simulink model "ANCwithError"  (R2023b)
settings: Solver=VariableStepAuto  StartTime=0.0  StopTime=10.0  RelTol=1e-3
libraries: matrix_library x54, dspadpt3 x30, raspberrypiAVlib x2, dspfdesign x2, audiosources x1
(part 1 of 2)
settings Model: Creator=aaron  LastModifiedBy=aaron

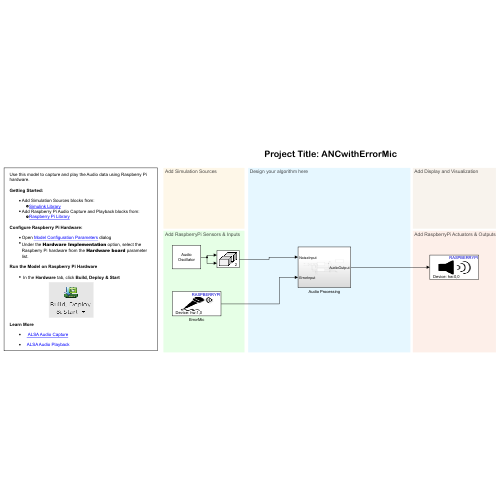
[thumbnail: Simulink's stored preview of the top-level diagram]
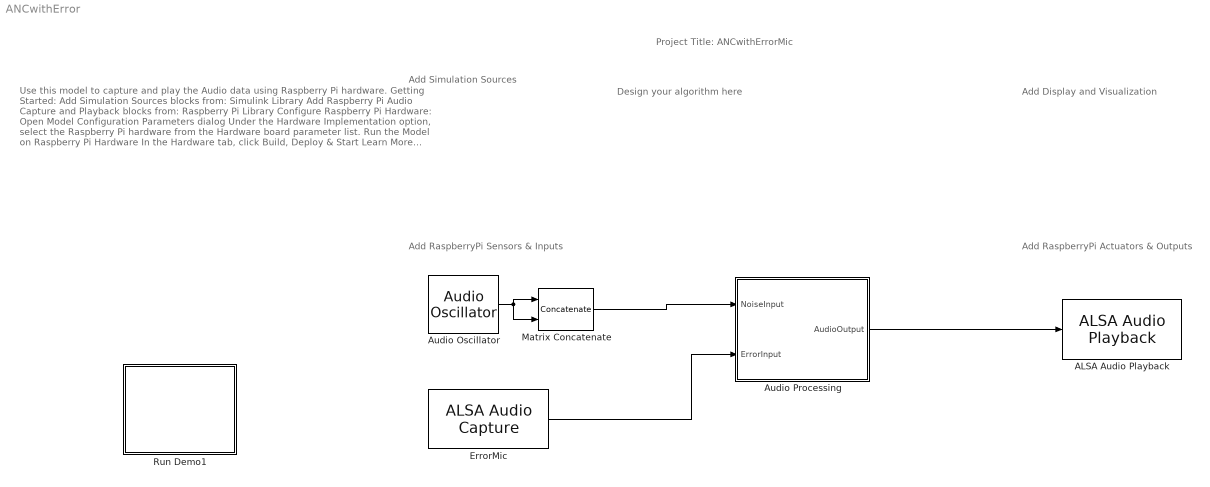
== system ANCwithError ==
  note: Use this model to capture and play the Audio data using Raspberry Pi hardware.
      |
      | Getting Started:
      |
      | Add Simulation Sources blocks from:
      | Simulink Library
      | Add Raspberry Pi Audio Capture and Playback blocks from:
      | Raspberry Pi Library
      |
      | Configure Raspberry Pi Hardware:
      |
      | Open Model Configuration Parameters dialog
      | Under the Hardware Implementation option, select the Raspberry Pi hardware from the Hardware board parameter list.
      |
      | Run the Model on Raspberry Pi Hardware
      |
      | In the Hardware tab, click Build, Deploy & Start
      |
      | Learn More
      | ALSA Audio Capture
      | ALSA Audio Playback
  note: Add Simulation Sources
  note: Add RaspberryPi Sensors & Inputs
  note: Project Title: ANCwithErrorMic
  note: Add Display and Visualization
  note: Add RaspberryPi Actuators & Outputs
  note: Design your algorithm here
  ALSA Audio Playback : raspberrypiAVlib/ALSA Audio Playback  deviceStr='hw:0,0'  sampleRateEnum=44100  queueDuration=0.5  blockPlatform=Raspberry Pi
  Audio Oscillator : audiosources/Audio Oscillator  FrequencyPort=off  Frequency=300  AmplitudePort=off  Amplitude=30000  DCOffsetPort=off  PhaseOffset=0  DCOffset=0  WidthPort=off  Width=1  DutyCyclePort=off  DutyCycle=0.5  SampsPerFrame=10  Fs=44100  OutputDataType=double  SimulateUsing=Code generation
      settings: SignalType=sine
  Audio Processing : Subsystem
  ErrorMic : raspberrypiAVlib/ALSA Audio Capture  deviceStr='hw:1,0'  DataBitDepth=16-bit integer  numberOfChannels=2  sampleRateEnum=44100  frameSize=SpF  QueueDuration=0.5  blockPlatform=Raspberry Pi
  Matrix Concatenate : Concatenate  Mode=Multidimensional array  ConcatenateDimension=2
  Run Demo1 : Subsystem  Description=Controls host-side RTDX processing.
      mask Display: pic=imread('raspberrypiBuildDeployAndStart.png');image(pic);
  wires:
  Matrix Concatenate/1 -> Audio Processing/1(NoiseInput)
  Audio Processing/1(AudioOutput) -> ALSA Audio Playback/1
  Audio Oscillator/1 -> Matrix Concatenate/2, Matrix Concatenate/1
  ErrorMic/1 -> Audio Processing/2(ErrorInput)

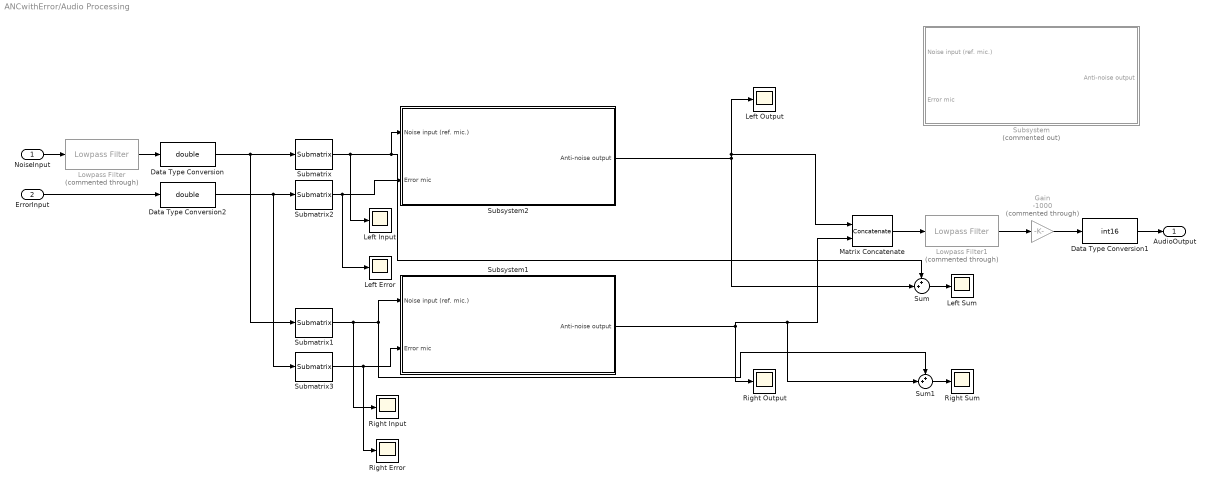
== system ANCwithError/Audio Processing ==
  NoiseInput : Inport
  ErrorInput : Inport  Port=2
  Data Type Conversion : DataTypeConversion  OutDataTypeStr=double  SaturateOnIntegerOverflow=off  RndMeth=Floor
  Data Type Conversion1 : DataTypeConversion  OutDataTypeStr=int16  SaturateOnIntegerOverflow=off  RndMeth=Floor  LockScale=on
  Data Type Conversion2 : DataTypeConversion  OutDataTypeStr=double  SaturateOnIntegerOverflow=off  RndMeth=Floor
  Gain : Gain  Commented=through  Gain=-1000
  Left Error : Scope
  Left Input : Scope
  Left Output : Scope
  Left Sum : Scope
  Lowpass Filter : dspfdesign/Lowpass Filter  Commented=through  FilterType=FIR  DesignForMinimumOrder=on  FilterOrder=50  PassbandFrequency=6e2  StopbandFrequency=10e2  PassbandRipple=0.1  StopbandAttenuation=80  SampleRateMode=Specify on dialog  SampleRate=44100  SimulateUsing=Interpreted execution  roundingMode=Floor  coeffsDataTypeStr=fixdt(1,16)
  Lowpass Filter1 : dspfdesign/Lowpass Filter  Commented=through  FilterType=FIR  DesignForMinimumOrder=on  FilterOrder=50  PassbandFrequency=6e2  StopbandFrequency=10e2  PassbandRipple=0.1  StopbandAttenuation=80  SampleRateMode=Specify on dialog  SampleRate=44100  SimulateUsing=Interpreted execution  roundingMode=Floor  coeffsDataTypeStr=fixdt(1,16)
  Matrix Concatenate : Concatenate  Mode=Multidimensional array  ConcatenateDimension=2
  Right Error : Scope
  Right Input : Scope
  Right Output : Scope
  Right Sum : Scope
  Submatrix : matrix_library/Submatrix  RowSpan=All rows  RowStartMode=First  RowStartIndex=1  RowEndMode=Last  RowEndIndex=1  ColSpan=One column  ColStartMode=First  ColStartIndex=1  ColEndMode=Last  ColEndIndex=1
  Submatrix1 : matrix_library/Submatrix  RowSpan=All rows  RowStartMode=First  RowStartIndex=1  RowEndMode=Last  RowEndIndex=1  ColSpan=One column  ColStartMode=Last  ColStartIndex=1  ColEndMode=Last  ColEndIndex=1
  Submatrix2 : matrix_library/Submatrix  RowSpan=All rows  RowStartMode=First  RowStartIndex=1  RowEndMode=Last  RowEndIndex=1  ColSpan=One column  ColStartMode=First  ColStartIndex=1  ColEndMode=Last  ColEndIndex=1
  Submatrix3 : matrix_library/Submatrix  RowSpan=All rows  RowStartMode=First  RowStartIndex=1  RowEndMode=Last  RowEndIndex=1  ColSpan=One column  ColStartMode=Last  ColStartIndex=1  ColEndMode=Last  ColEndIndex=1
  Subsystem : Subsystem  Commented=on  TreatAsAtomicUnit=on
  Subsystem1 : Subsystem  TreatAsAtomicUnit=on
  Subsystem2 : Subsystem  TreatAsAtomicUnit=on
  Sum : Sum  Inputs=++|
  Sum1 : Sum  Inputs=++|
  AudioOutput : Outport
  wires:
  Data Type Conversion/1 -> Submatrix1/1, Submatrix/1
  Submatrix/1 -> Subsystem2/1(Noise input (ref. mic.)), Sum/1, Left Input/1
  NoiseInput/1 -> Lowpass Filter/1
  Submatrix1/1 -> Sum1/1, Subsystem1/1(Noise input (ref. mic.)), Right Input/1
  Subsystem1/1(Anti-noise output) -> Sum1/2, Matrix Concatenate/2, Right Output/1
  Lowpass Filter/1 -> Data Type Conversion/1
  Gain/1 -> Data Type Conversion1/1
  Lowpass Filter1/1 -> Gain/1
  Data Type Conversion1/1 -> AudioOutput/1
  Matrix Concatenate/1 -> Lowpass Filter1/1
  Sum1/1 -> Right Sum/1
  Subsystem2/1(Anti-noise output) -> Left Output/1, Matrix Concatenate/1, Sum/2
  Sum/1 -> Left Sum/1
  ErrorInput/1 -> Data Type Conversion2/1
  Data Type Conversion2/1 -> Submatrix3/1, Submatrix2/1
  Submatrix2/1 -> Left Error/1, Subsystem2/2(Error mic)
  Submatrix3/1 -> Right Error/1, Subsystem1/2(Error mic)

== system ANCwithError/Run Demo1 ==

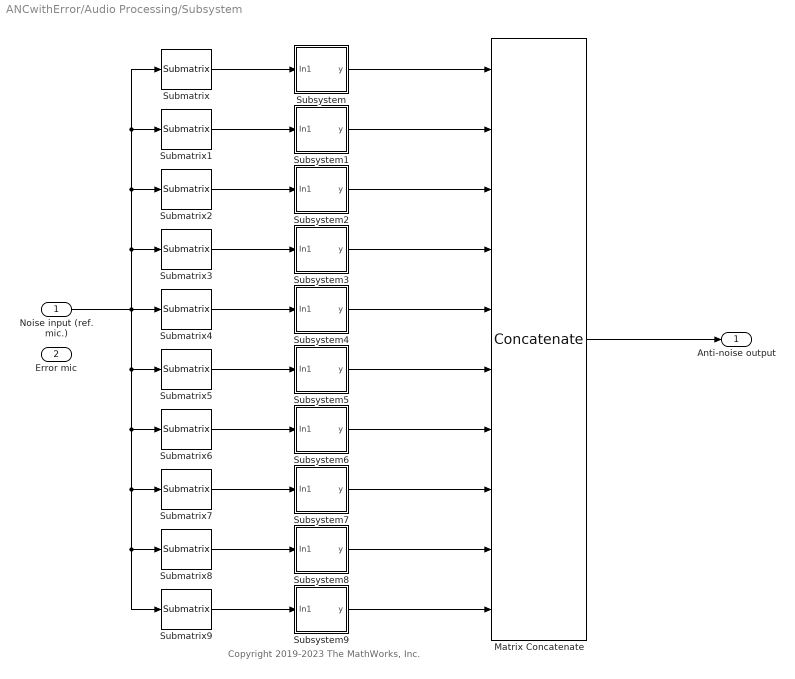
== system ANCwithError/Audio Processing/Subsystem ==
  note: Copyright 2019-2023 The MathWorks, Inc.
  Noise input (ref. mic.) : Inport
  Error mic : Inport  Port=2
  Matrix Concatenate : Concatenate  NumInputs=10  Mode=Multidimensional array
  Submatrix : matrix_library/Submatrix  RowSpan=One row  RowStartMode=Index  RowStartIndex=1  RowEndMode=Last  RowEndIndex=1  ColSpan=One column  ColStartMode=First  ColStartIndex=1  ColEndMode=Last  ColEndIndex=1
  Submatrix1 : matrix_library/Submatrix  RowSpan=One row  RowStartMode=Index  RowStartIndex=2  RowEndMode=Last  RowEndIndex=1  ColSpan=One column  ColStartMode=First  ColStartIndex=1  ColEndMode=Last  ColEndIndex=1
  Submatrix2 : matrix_library/Submatrix  RowSpan=One row  RowStartMode=Index  RowStartIndex=3  RowEndMode=Last  RowEndIndex=1  ColSpan=One column  ColStartMode=First  ColStartIndex=1  ColEndMode=Last  ColEndIndex=1
  Submatrix3 : matrix_library/Submatrix  RowSpan=One row  RowStartMode=Index  RowStartIndex=4  RowEndMode=Last  RowEndIndex=1  ColSpan=One column  ColStartMode=First  ColStartIndex=1  ColEndMode=Last  ColEndIndex=1
  Submatrix4 : matrix_library/Submatrix  RowSpan=One row  RowStartMode=Index  RowStartIndex=5  RowEndMode=Last  RowEndIndex=1  ColSpan=One column  ColStartMode=First  ColStartIndex=1  ColEndMode=Last  ColEndIndex=1
  Submatrix5 : matrix_library/Submatrix  RowSpan=One row  RowStartMode=Index  RowStartIndex=6  RowEndMode=Last  RowEndIndex=1  ColSpan=One column  ColStartMode=First  ColStartIndex=1  ColEndMode=Last  ColEndIndex=1
  Submatrix6 : matrix_library/Submatrix  RowSpan=One row  RowStartMode=Index  RowStartIndex=7  RowEndMode=Last  RowEndIndex=1  ColSpan=One column  ColStartMode=First  ColStartIndex=1  ColEndMode=Last  ColEndIndex=1
  Submatrix7 : matrix_library/Submatrix  RowSpan=One row  RowStartMode=Index  RowStartIndex=8  RowEndMode=Last  RowEndIndex=1  ColSpan=One column  ColStartMode=First  ColStartIndex=1  ColEndMode=Last  ColEndIndex=1
  Submatrix8 : matrix_library/Submatrix  RowSpan=One row  RowStartMode=Index  RowStartIndex=9  RowEndMode=Last  RowEndIndex=1  ColSpan=One column  ColStartMode=First  ColStartIndex=1  ColEndMode=Last  ColEndIndex=1
  Submatrix9 : matrix_library/Submatrix  RowSpan=One row  RowStartMode=Index  RowStartIndex=10  RowEndMode=Last  RowEndIndex=1  ColSpan=One column  ColStartMode=First  ColStartIndex=1  ColEndMode=Last  ColEndIndex=1
  Subsystem : Subsystem
  Subsystem1 : Subsystem
  Subsystem2 : Subsystem
  Subsystem3 : Subsystem
  Subsystem4 : Subsystem
  Subsystem5 : Subsystem
  Subsystem6 : Subsystem
  Subsystem7 : Subsystem
  Subsystem8 : Subsystem
  Subsystem9 : Subsystem
  Anti-noise output : Outport
  wires:
  Submatrix1/1 -> Subsystem1/1(In1)
  Submatrix2/1 -> Subsystem2/1(In1)
  Submatrix3/1 -> Subsystem3/1(In1)
  Submatrix4/1 -> Subsystem4/1(In1)
  Submatrix5/1 -> Subsystem5/1(In1)
  Submatrix6/1 -> Subsystem6/1(In1)
  Submatrix7/1 -> Subsystem7/1(In1)
  Submatrix8/1 -> Subsystem8/1(In1)
  Submatrix9/1 -> Subsystem9/1(In1)
  Noise input (ref. mic.)/1 -> Submatrix9/1, Submatrix8/1, Submatrix7/1, Submatrix6/1, Submatrix5/1, Submatrix/1, Submatrix1/1, Submatrix2/1, Submatrix3/1, Submatrix4/1
  Subsystem1/1(y) -> Matrix Concatenate/2
  Subsystem2/1(y) -> Matrix Concatenate/3
  Subsystem3/1(y) -> Matrix Concatenate/4
  Subsystem4/1(y) -> Matrix Concatenate/5
  Subsystem5/1(y) -> Matrix Concatenate/6
  Matrix Concatenate/1 -> Anti-noise output/1
  Subsystem6/1(y) -> Matrix Concatenate/7
  Subsystem7/1(y) -> Matrix Concatenate/8
  Subsystem8/1(y) -> Matrix Concatenate/9
  Subsystem9/1(y) -> Matrix Concatenate/10
  Submatrix/1 -> Subsystem/1(In1)
  Subsystem/1(y) -> Matrix Concatenate/1

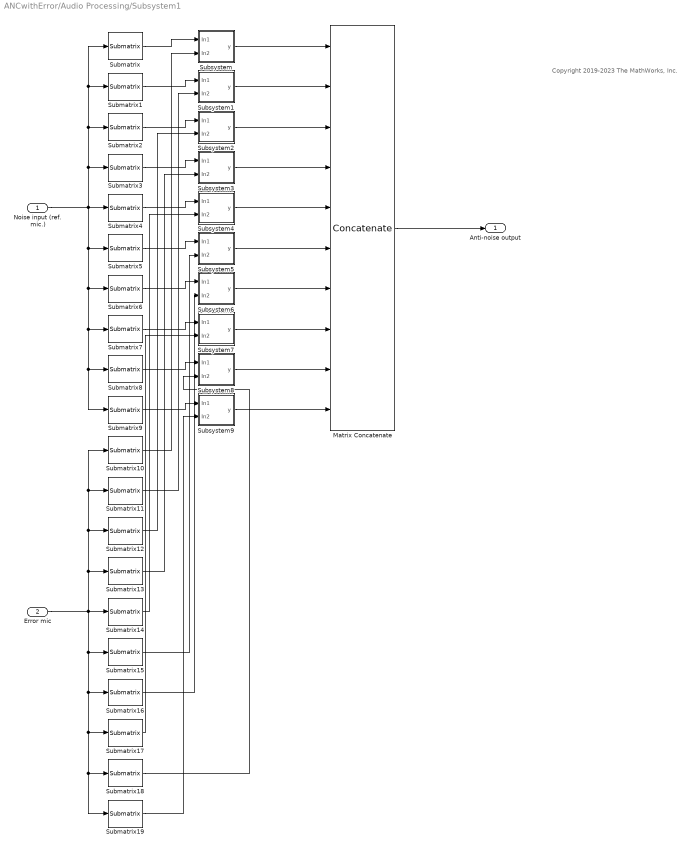
== system ANCwithError/Audio Processing/Subsystem1 ==
  note: Copyright 2019-2023 The MathWorks, Inc.
  Noise input (ref. mic.) : Inport
  Error mic : Inport  Port=2
  Matrix Concatenate : Concatenate  NumInputs=10  Mode=Multidimensional array
  Submatrix : matrix_library/Submatrix  RowSpan=One row  RowStartMode=Index  RowStartIndex=1  RowEndMode=Last  RowEndIndex=1  ColSpan=One column  ColStartMode=First  ColStartIndex=1  ColEndMode=Last  ColEndIndex=1
  Submatrix1 : matrix_library/Submatrix  RowSpan=One row  RowStartMode=Index  RowStartIndex=2  RowEndMode=Last  RowEndIndex=1  ColSpan=One column  ColStartMode=First  ColStartIndex=1  ColEndMode=Last  ColEndIndex=1
  Submatrix10 : matrix_library/Submatrix  RowSpan=One row  RowStartMode=Index  RowStartIndex=1  RowEndMode=Last  RowEndIndex=1  ColSpan=One column  ColStartMode=First  ColStartIndex=1  ColEndMode=Last  ColEndIndex=1
  Submatrix11 : matrix_library/Submatrix  RowSpan=One row  RowStartMode=Index  RowStartIndex=2  RowEndMode=Last  RowEndIndex=1  ColSpan=One column  ColStartMode=First  ColStartIndex=1  ColEndMode=Last  ColEndIndex=1
  Submatrix12 : matrix_library/Submatrix  RowSpan=One row  RowStartMode=Index  RowStartIndex=3  RowEndMode=Last  RowEndIndex=1  ColSpan=One column  ColStartMode=First  ColStartIndex=1  ColEndMode=Last  ColEndIndex=1
  Submatrix13 : matrix_library/Submatrix  RowSpan=One row  RowStartMode=Index  RowStartIndex=4  RowEndMode=Last  RowEndIndex=1  ColSpan=One column  ColStartMode=First  ColStartIndex=1  ColEndMode=Last  ColEndIndex=1
  Submatrix14 : matrix_library/Submatrix  RowSpan=One row  RowStartMode=Index  RowStartIndex=5  RowEndMode=Last  RowEndIndex=1  ColSpan=One column  ColStartMode=First  ColStartIndex=1  ColEndMode=Last  ColEndIndex=1
  Submatrix15 : matrix_library/Submatrix  RowSpan=One row  RowStartMode=Index  RowStartIndex=6  RowEndMode=Last  RowEndIndex=1  ColSpan=One column  ColStartMode=First  ColStartIndex=1  ColEndMode=Last  ColEndIndex=1
  Submatrix16 : matrix_library/Submatrix  RowSpan=One row  RowStartMode=Index  RowStartIndex=7  RowEndMode=Last  RowEndIndex=1  ColSpan=One column  ColStartMode=First  ColStartIndex=1  ColEndMode=Last  ColEndIndex=1
  Submatrix17 : matrix_library/Submatrix  RowSpan=One row  RowStartMode=Index  RowStartIndex=8  RowEndMode=Last  RowEndIndex=1  ColSpan=One column  ColStartMode=First  ColStartIndex=1  ColEndMode=Last  ColEndIndex=1
  Submatrix18 : matrix_library/Submatrix  RowSpan=One row  RowStartMode=Index  RowStartIndex=9  RowEndMode=Last  RowEndIndex=1  ColSpan=One column  ColStartMode=First  ColStartIndex=1  ColEndMode=Last  ColEndIndex=1
  Submatrix19 : matrix_library/Submatrix  RowSpan=One row  RowStartMode=Index  RowStartIndex=10  RowEndMode=Last  RowEndIndex=1  ColSpan=One column  ColStartMode=First  ColStartIndex=1  ColEndMode=Last  ColEndIndex=1
  Submatrix2 : matrix_library/Submatrix  RowSpan=One row  RowStartMode=Index  RowStartIndex=3  RowEndMode=Last  RowEndIndex=1  ColSpan=One column  ColStartMode=First  ColStartIndex=1  ColEndMode=Last  ColEndIndex=1
  Submatrix3 : matrix_library/Submatrix  RowSpan=One row  RowStartMode=Index  RowStartIndex=4  RowEndMode=Last  RowEndIndex=1  ColSpan=One column  ColStartMode=First  ColStartIndex=1  ColEndMode=Last  ColEndIndex=1
  Submatrix4 : matrix_library/Submatrix  RowSpan=One row  RowStartMode=Index  RowStartIndex=5  RowEndMode=Last  RowEndIndex=1  ColSpan=One column  ColStartMode=First  ColStartIndex=1  ColEndMode=Last  ColEndIndex=1
  Submatrix5 : matrix_library/Submatrix  RowSpan=One row  RowStartMode=Index  RowStartIndex=6  RowEndMode=Last  RowEndIndex=1  ColSpan=One column  ColStartMode=First  ColStartIndex=1  ColEndMode=Last  ColEndIndex=1
  Submatrix6 : matrix_library/Submatrix  RowSpan=One row  RowStartMode=Index  RowStartIndex=7  RowEndMode=Last  RowEndIndex=1  ColSpan=One column  ColStartMode=First  ColStartIndex=1  ColEndMode=Last  ColEndIndex=1
  Submatrix7 : matrix_library/Submatrix  RowSpan=One row  RowStartMode=Index  RowStartIndex=8  RowEndMode=Last  RowEndIndex=1  ColSpan=One column  ColStartMode=First  ColStartIndex=1  ColEndMode=Last  ColEndIndex=1
  Submatrix8 : matrix_library/Submatrix  RowSpan=One row  RowStartMode=Index  RowStartIndex=9  RowEndMode=Last  RowEndIndex=1  ColSpan=One column  ColStartMode=First  ColStartIndex=1  ColEndMode=Last  ColEndIndex=1
  Submatrix9 : matrix_library/Submatrix  RowSpan=One row  RowStartMode=Index  RowStartIndex=10  RowEndMode=Last  RowEndIndex=1  ColSpan=One column  ColStartMode=First  ColStartIndex=1  ColEndMode=Last  ColEndIndex=1
  Subsystem : Subsystem
  Subsystem1 : Subsystem
  Subsystem2 : Subsystem
  Subsystem3 : Subsystem
  Subsystem4 : Subsystem
  Subsystem5 : Subsystem
  Subsystem6 : Subsystem
  Subsystem7 : Subsystem
  Subsystem8 : Subsystem
  Subsystem9 : Subsystem
  Anti-noise output : Outport
  wires:
  Submatrix1/1 -> Subsystem1/1(In1)
  Submatrix2/1 -> Subsystem2/1(In1)
  Submatrix3/1 -> Subsystem3/1(In1)
  Submatrix4/1 -> Subsystem4/1(In1)
  Submatrix5/1 -> Subsystem5/1(In1)
  Submatrix6/1 -> Subsystem6/1(In1)
  Submatrix7/1 -> Subsystem7/1(In1)
  Submatrix8/1 -> Subsystem8/1(In1)
  Submatrix9/1 -> Subsystem9/1(In1)
  Noise input (ref. mic.)/1 -> Submatrix9/1, Submatrix8/1, Submatrix7/1, Submatrix6/1, Submatrix5/1, Submatrix/1, Submatrix1/1, Submatrix2/1, Submatrix3/1, Submatrix4/1
  Subsystem1/1(y) -> Matrix Concatenate/2
  Subsystem2/1(y) -> Matrix Concatenate/3
  Subsystem3/1(y) -> Matrix Concatenate/4
  Subsystem4/1(y) -> Matrix Concatenate/5
  Subsystem5/1(y) -> Matrix Concatenate/6
  Matrix Concatenate/1 -> Anti-noise output/1
  Subsystem6/1(y) -> Matrix Concatenate/7
  Subsystem7/1(y) -> Matrix Concatenate/8
  Subsystem8/1(y) -> Matrix Concatenate/9
  Subsystem9/1(y) -> Matrix Concatenate/10
  Submatrix/1 -> Subsystem/1(In1)
  Subsystem/1(y) -> Matrix Concatenate/1
  Error mic/1 -> Submatrix19/1, Submatrix18/1, Submatrix17/1, Submatrix16/1, Submatrix15/1, Submatrix10/1, Submatrix11/1, Submatrix12/1, Submatrix13/1, Submatrix14/1
  Submatrix10/1 -> Subsystem/2(In2)
  Submatrix11/1 -> Subsystem1/2(In2)
  Submatrix12/1 -> Subsystem2/2(In2)
  Submatrix13/1 -> Subsystem3/2(In2)
  Submatrix14/1 -> Subsystem4/2(In2)
  Submatrix15/1 -> Subsystem5/2(In2)
  Submatrix16/1 -> Subsystem6/2(In2)
  Submatrix17/1 -> Subsystem7/2(In2)
  Submatrix18/1 -> Subsystem8/2(In2)
  Submatrix19/1 -> Subsystem9/2(In2)

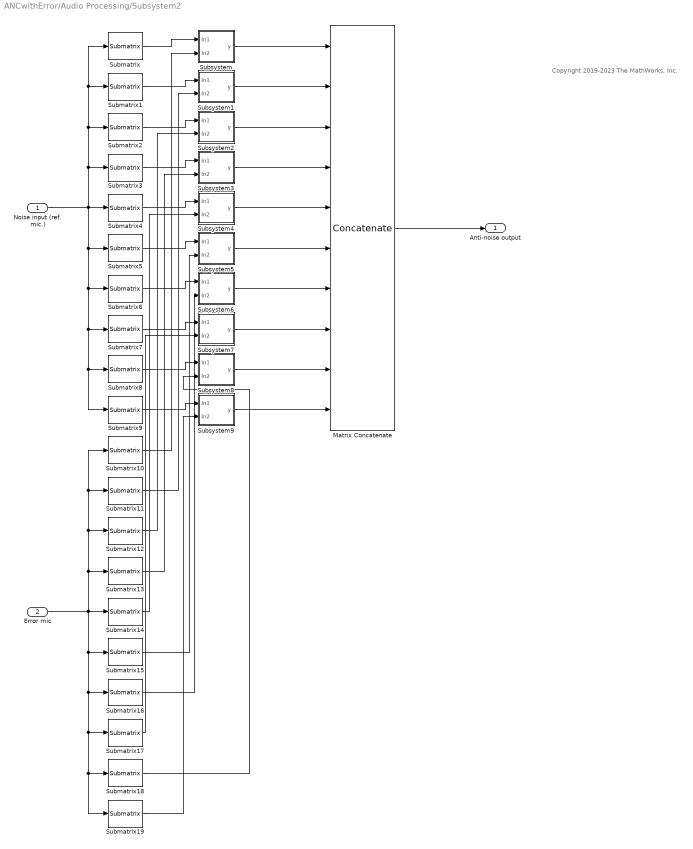
== system ANCwithError/Audio Processing/Subsystem2 ==
  note: Copyright 2019-2023 The MathWorks, Inc.
  Noise input (ref. mic.) : Inport
  Error mic : Inport  Port=2
  Matrix Concatenate : Concatenate  NumInputs=10  Mode=Multidimensional array
  Submatrix : matrix_library/Submatrix  RowSpan=One row  RowStartMode=Index  RowStartIndex=1  RowEndMode=Last  RowEndIndex=1  ColSpan=One column  ColStartMode=First  ColStartIndex=1  ColEndMode=Last  ColEndIndex=1
  Submatrix1 : matrix_library/Submatrix  RowSpan=One row  RowStartMode=Index  RowStartIndex=2  RowEndMode=Last  RowEndIndex=1  ColSpan=One column  ColStartMode=First  ColStartIndex=1  ColEndMode=Last  ColEndIndex=1
  Submatrix10 : matrix_library/Submatrix  RowSpan=One row  RowStartMode=Index  RowStartIndex=1  RowEndMode=Last  RowEndIndex=1  ColSpan=One column  ColStartMode=First  ColStartIndex=1  ColEndMode=Last  ColEndIndex=1
  Submatrix11 : matrix_library/Submatrix  RowSpan=One row  RowStartMode=Index  RowStartIndex=2  RowEndMode=Last  RowEndIndex=1  ColSpan=One column  ColStartMode=First  ColStartIndex=1  ColEndMode=Last  ColEndIndex=1
  Submatrix12 : matrix_library/Submatrix  RowSpan=One row  RowStartMode=Index  RowStartIndex=3  RowEndMode=Last  RowEndIndex=1  ColSpan=One column  ColStartMode=First  ColStartIndex=1  ColEndMode=Last  ColEndIndex=1
  Submatrix13 : matrix_library/Submatrix  RowSpan=One row  RowStartMode=Index  RowStartIndex=4  RowEndMode=Last  RowEndIndex=1  ColSpan=One column  ColStartMode=First  ColStartIndex=1  ColEndMode=Last  ColEndIndex=1
  Submatrix14 : matrix_library/Submatrix  RowSpan=One row  RowStartMode=Index  RowStartIndex=5  RowEndMode=Last  RowEndIndex=1  ColSpan=One column  ColStartMode=First  ColStartIndex=1  ColEndMode=Last  ColEndIndex=1
  Submatrix15 : matrix_library/Submatrix  RowSpan=One row  RowStartMode=Index  RowStartIndex=6  RowEndMode=Last  RowEndIndex=1  ColSpan=One column  ColStartMode=First  ColStartIndex=1  ColEndMode=Last  ColEndIndex=1
  Submatrix16 : matrix_library/Submatrix  RowSpan=One row  RowStartMode=Index  RowStartIndex=7  RowEndMode=Last  RowEndIndex=1  ColSpan=One column  ColStartMode=First  ColStartIndex=1  ColEndMode=Last  ColEndIndex=1
  Submatrix17 : matrix_library/Submatrix  RowSpan=One row  RowStartMode=Index  RowStartIndex=8  RowEndMode=Last  RowEndIndex=1  ColSpan=One column  ColStartMode=First  ColStartIndex=1  ColEndMode=Last  ColEndIndex=1
  Submatrix18 : matrix_library/Submatrix  RowSpan=One row  RowStartMode=Index  RowStartIndex=9  RowEndMode=Last  RowEndIndex=1  ColSpan=One column  ColStartMode=First  ColStartIndex=1  ColEndMode=Last  ColEndIndex=1
  Submatrix19 : matrix_library/Submatrix  RowSpan=One row  RowStartMode=Index  RowStartIndex=10  RowEndMode=Last  RowEndIndex=1  ColSpan=One column  ColStartMode=First  ColStartIndex=1  ColEndMode=Last  ColEndIndex=1
  Submatrix2 : matrix_library/Submatrix  RowSpan=One row  RowStartMode=Index  RowStartIndex=3  RowEndMode=Last  RowEndIndex=1  ColSpan=One column  ColStartMode=First  ColStartIndex=1  ColEndMode=Last  ColEndIndex=1
  Submatrix3 : matrix_library/Submatrix  RowSpan=One row  RowStartMode=Index  RowStartIndex=4  RowEndMode=Last  RowEndIndex=1  ColSpan=One column  ColStartMode=First  ColStartIndex=1  ColEndMode=Last  ColEndIndex=1
  Submatrix4 : matrix_library/Submatrix  RowSpan=One row  RowStartMode=Index  RowStartIndex=5  RowEndMode=Last  RowEndIndex=1  ColSpan=One column  ColStartMode=First  ColStartIndex=1  ColEndMode=Last  ColEndIndex=1
  Submatrix5 : matrix_library/Submatrix  RowSpan=One row  RowStartMode=Index  RowStartIndex=6  RowEndMode=Last  RowEndIndex=1  ColSpan=One column  ColStartMode=First  ColStartIndex=1  ColEndMode=Last  ColEndIndex=1
  Submatrix6 : matrix_library/Submatrix  RowSpan=One row  RowStartMode=Index  RowStartIndex=7  RowEndMode=Last  RowEndIndex=1  ColSpan=One column  ColStartMode=First  ColStartIndex=1  ColEndMode=Last  ColEndIndex=1
  Submatrix7 : matrix_library/Submatrix  RowSpan=One row  RowStartMode=Index  RowStartIndex=8  RowEndMode=Last  RowEndIndex=1  ColSpan=One column  ColStartMode=First  ColStartIndex=1  ColEndMode=Last  ColEndIndex=1
  Submatrix8 : matrix_library/Submatrix  RowSpan=One row  RowStartMode=Index  RowStartIndex=9  RowEndMode=Last  RowEndIndex=1  ColSpan=One column  ColStartMode=First  ColStartIndex=1  ColEndMode=Last  ColEndIndex=1
  Submatrix9 : matrix_library/Submatrix  RowSpan=One row  RowStartMode=Index  RowStartIndex=10  RowEndMode=Last  RowEndIndex=1  ColSpan=One column  ColStartMode=First  ColStartIndex=1  ColEndMode=Last  ColEndIndex=1
  Subsystem : Subsystem
  Subsystem1 : Subsystem
  Subsystem2 : Subsystem
  Subsystem3 : Subsystem
  Subsystem4 : Subsystem
  Subsystem5 : Subsystem
  Subsystem6 : Subsystem
  Subsystem7 : Subsystem
  Subsystem8 : Subsystem
  Subsystem9 : Subsystem
  Anti-noise output : Outport
  wires:
  Submatrix1/1 -> Subsystem1/1(In1)
  Submatrix2/1 -> Subsystem2/1(In1)
  Submatrix3/1 -> Subsystem3/1(In1)
  Submatrix4/1 -> Subsystem4/1(In1)
  Submatrix5/1 -> Subsystem5/1(In1)
  Submatrix6/1 -> Subsystem6/1(In1)
  Submatrix7/1 -> Subsystem7/1(In1)
  Submatrix8/1 -> Subsystem8/1(In1)
  Submatrix9/1 -> Subsystem9/1(In1)
  Noise input (ref. mic.)/1 -> Submatrix9/1, Submatrix8/1, Submatrix7/1, Submatrix6/1, Submatrix5/1, Submatrix/1, Submatrix1/1, Submatrix2/1, Submatrix3/1, Submatrix4/1
  Subsystem1/1(y) -> Matrix Concatenate/2
  Subsystem2/1(y) -> Matrix Concatenate/3
  Subsystem3/1(y) -> Matrix Concatenate/4
  Subsystem4/1(y) -> Matrix Concatenate/5
  Subsystem5/1(y) -> Matrix Concatenate/6
  Matrix Concatenate/1 -> Anti-noise output/1
  Subsystem6/1(y) -> Matrix Concatenate/7
  Subsystem7/1(y) -> Matrix Concatenate/8
  Subsystem8/1(y) -> Matrix Concatenate/9
  Subsystem9/1(y) -> Matrix Concatenate/10
  Submatrix/1 -> Subsystem/1(In1)
  Subsystem/1(y) -> Matrix Concatenate/1
  Error mic/1 -> Submatrix19/1, Submatrix18/1, Submatrix17/1, Submatrix16/1, Submatrix15/1, Submatrix10/1, Submatrix11/1, Submatrix12/1, Submatrix13/1, Submatrix14/1
  Submatrix10/1 -> Subsystem/2(In2)
  Submatrix11/1 -> Subsystem1/2(In2)
  Submatrix12/1 -> Subsystem2/2(In2)
  Submatrix13/1 -> Subsystem3/2(In2)
  Submatrix14/1 -> Subsystem4/2(In2)
  Submatrix15/1 -> Subsystem5/2(In2)
  Submatrix16/1 -> Subsystem6/2(In2)
  Submatrix17/1 -> Subsystem7/2(In2)
  Submatrix18/1 -> Subsystem8/2(In2)
  Submatrix19/1 -> Subsystem9/2(In2)

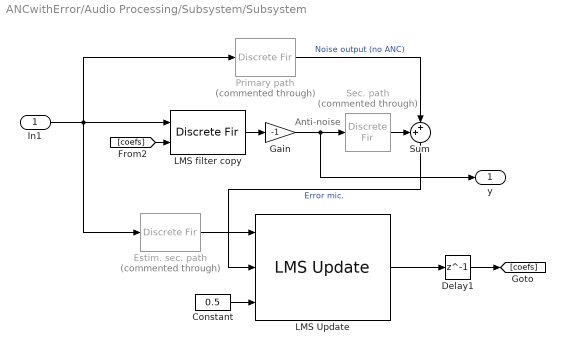
== system ANCwithError/Audio Processing/Subsystem/Subsystem ==
  note: Anti-noise
  In1 : Inport
  Constant : Constant  Value=0.5
  Delay1 : Delay  DelayLength=1
  Estim. sec. path : DiscreteFir  Commented=through  Coefficients="[0.466  0.533  -0.257  -0.274  -0.231  -0.175]"
  Gain : Gain  Gain=-1
  LMS Update : dspadpt3/LMS Update  Method=Normalized LMS  Length=200  NumFilters=1  StepSizeSource=Input port  StepSize=0.1  LeakageFactor=1.0  InitialConditions=0  AdaptiveFilterMode=Tapped delay-line FIR filter  EnableAdaptInput=off  EnableResetInput=off  SimulateUsing=Interpreted execution
  LMS filter copy : DiscreteFir  CoefSource=Input port
      settings: InputPortMap=u0,u1
  Primary path : DiscreteFir  Commented=through  Coefficients=conv([0.5 0.5 -.3 -.3 -.2 -.2],[.1 -.1 .2 -.2 .3 -.3 .15 -.15])
  Sec. path : DiscreteFir  Commented=through  Coefficients=[0.5 0.5 -.3 -.3 -.2 -.2]
  Sum : Sum  Inputs=++|
  y : Outport
  wires:
  Primary path/1 -> Sum/2  "Noise output (no ANC)"
  Gain/1 -> y/1, Sec. path/1
  Constant/1 -> LMS Update/3
  LMS filter copy/1 -> Gain/1
  [coefs] -> LMS filter copy/2
  Sum/1 -> LMS Update/2  "Error mic."
  Delay1/1 -> [coefs]
  LMS Update/1 -> Delay1/1
  In1/1 -> Primary path/1, Estim. sec. path/1, LMS filter copy/1
  Estim. sec. path/1 -> LMS Update/1
  Sec. path/1 -> Sum/1

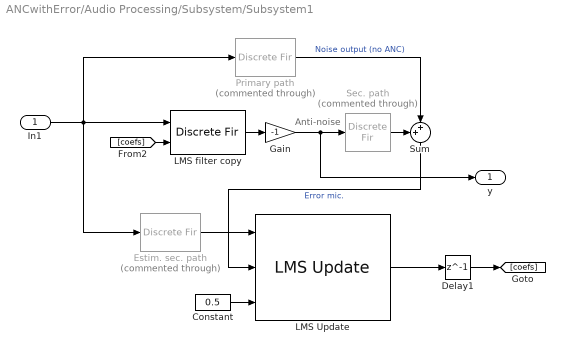
== system ANCwithError/Audio Processing/Subsystem/Subsystem1 ==
  note: Anti-noise
  In1 : Inport
  Constant : Constant  Value=0.5
  Delay1 : Delay  DelayLength=1
  Estim. sec. path : DiscreteFir  Commented=through  Coefficients="[0.466  0.533  -0.257  -0.274  -0.231  -0.175]"
  Gain : Gain  Gain=-1
  LMS Update : dspadpt3/LMS Update  Method=Normalized LMS  Length=200  NumFilters=1  StepSizeSource=Input port  StepSize=0.1  LeakageFactor=1.0  InitialConditions=0  AdaptiveFilterMode=Tapped delay-line FIR filter  EnableAdaptInput=off  EnableResetInput=off  SimulateUsing=Interpreted execution
  LMS filter copy : DiscreteFir  CoefSource=Input port
      settings: InputPortMap=u0,u1
  Primary path : DiscreteFir  Commented=through  Coefficients=conv([0.5 0.5 -.3 -.3 -.2 -.2],[.1 -.1 .2 -.2 .3 -.3 .15 -.15])
  Sec. path : DiscreteFir  Commented=through  Coefficients=[0.5 0.5 -.3 -.3 -.2 -.2]
  Sum : Sum  Inputs=++|
  y : Outport
  wires:
  Primary path/1 -> Sum/2  "Noise output (no ANC)"
  Gain/1 -> y/1, Sec. path/1
  Constant/1 -> LMS Update/3
  LMS filter copy/1 -> Gain/1
  [coefs] -> LMS filter copy/2
  Sum/1 -> LMS Update/2  "Error mic."
  Delay1/1 -> [coefs]
  LMS Update/1 -> Delay1/1
  In1/1 -> Primary path/1, Estim. sec. path/1, LMS filter copy/1
  Estim. sec. path/1 -> LMS Update/1
  Sec. path/1 -> Sum/1

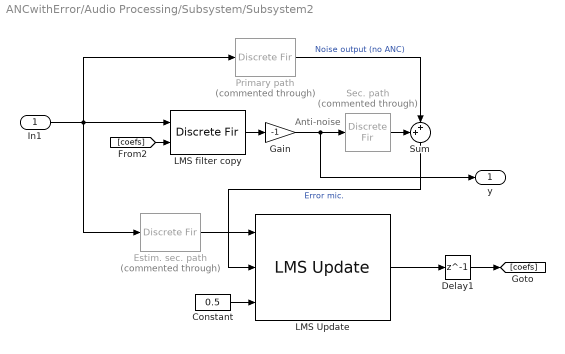
== system ANCwithError/Audio Processing/Subsystem/Subsystem2 ==
  note: Anti-noise
  In1 : Inport
  Constant : Constant  Value=0.5
  Delay1 : Delay  DelayLength=1
  Estim. sec. path : DiscreteFir  Commented=through  Coefficients="[0.466  0.533  -0.257  -0.274  -0.231  -0.175]"
  Gain : Gain  Gain=-1
  LMS Update : dspadpt3/LMS Update  Method=Normalized LMS  Length=200  NumFilters=1  StepSizeSource=Input port  StepSize=0.1  LeakageFactor=1.0  InitialConditions=0  AdaptiveFilterMode=Tapped delay-line FIR filter  EnableAdaptInput=off  EnableResetInput=off  SimulateUsing=Interpreted execution
  LMS filter copy : DiscreteFir  CoefSource=Input port
      settings: InputPortMap=u0,u1
  Primary path : DiscreteFir  Commented=through  Coefficients=conv([0.5 0.5 -.3 -.3 -.2 -.2],[.1 -.1 .2 -.2 .3 -.3 .15 -.15])
  Sec. path : DiscreteFir  Commented=through  Coefficients=[0.5 0.5 -.3 -.3 -.2 -.2]
  Sum : Sum  Inputs=++|
  y : Outport
  wires:
  Primary path/1 -> Sum/2  "Noise output (no ANC)"
  Gain/1 -> y/1, Sec. path/1
  Constant/1 -> LMS Update/3
  LMS filter copy/1 -> Gain/1
  [coefs] -> LMS filter copy/2
  Sum/1 -> LMS Update/2  "Error mic."
  Delay1/1 -> [coefs]
  LMS Update/1 -> Delay1/1
  In1/1 -> Primary path/1, Estim. sec. path/1, LMS filter copy/1
  Estim. sec. path/1 -> LMS Update/1
  Sec. path/1 -> Sum/1

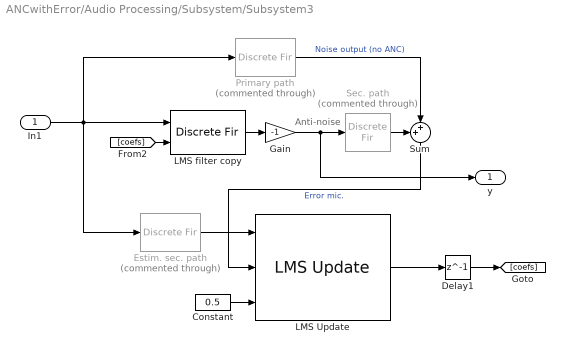
== system ANCwithError/Audio Processing/Subsystem/Subsystem3 ==
  note: Anti-noise
  In1 : Inport
  Constant : Constant  Value=0.5
  Delay1 : Delay  DelayLength=1
  Estim. sec. path : DiscreteFir  Commented=through  Coefficients="[0.466  0.533  -0.257  -0.274  -0.231  -0.175]"
  Gain : Gain  Gain=-1
  LMS Update : dspadpt3/LMS Update  Method=Normalized LMS  Length=200  NumFilters=1  StepSizeSource=Input port  StepSize=0.1  LeakageFactor=1.0  InitialConditions=0  AdaptiveFilterMode=Tapped delay-line FIR filter  EnableAdaptInput=off  EnableResetInput=off  SimulateUsing=Interpreted execution
  LMS filter copy : DiscreteFir  CoefSource=Input port
      settings: InputPortMap=u0,u1
  Primary path : DiscreteFir  Commented=through  Coefficients=conv([0.5 0.5 -.3 -.3 -.2 -.2],[.1 -.1 .2 -.2 .3 -.3 .15 -.15])
  Sec. path : DiscreteFir  Commented=through  Coefficients=[0.5 0.5 -.3 -.3 -.2 -.2]
  Sum : Sum  Inputs=++|
  y : Outport
  wires:
  Primary path/1 -> Sum/2  "Noise output (no ANC)"
  Gain/1 -> y/1, Sec. path/1
  Constant/1 -> LMS Update/3
  LMS filter copy/1 -> Gain/1
  [coefs] -> LMS filter copy/2
  Sum/1 -> LMS Update/2  "Error mic."
  Delay1/1 -> [coefs]
  LMS Update/1 -> Delay1/1
  In1/1 -> Primary path/1, Estim. sec. path/1, LMS filter copy/1
  Estim. sec. path/1 -> LMS Update/1
  Sec. path/1 -> Sum/1

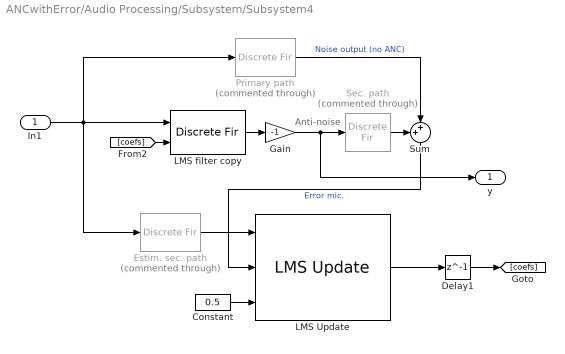
== system ANCwithError/Audio Processing/Subsystem/Subsystem4 ==
  note: Anti-noise
  In1 : Inport
  Constant : Constant  Value=0.5
  Delay1 : Delay  DelayLength=1
  Estim. sec. path : DiscreteFir  Commented=through  Coefficients="[0.466  0.533  -0.257  -0.274  -0.231  -0.175]"
  Gain : Gain  Gain=-1
  LMS Update : dspadpt3/LMS Update  Method=Normalized LMS  Length=200  NumFilters=1  StepSizeSource=Input port  StepSize=0.1  LeakageFactor=1.0  InitialConditions=0  AdaptiveFilterMode=Tapped delay-line FIR filter  EnableAdaptInput=off  EnableResetInput=off  SimulateUsing=Interpreted execution
  LMS filter copy : DiscreteFir  CoefSource=Input port
      settings: InputPortMap=u0,u1
  Primary path : DiscreteFir  Commented=through  Coefficients=conv([0.5 0.5 -.3 -.3 -.2 -.2],[.1 -.1 .2 -.2 .3 -.3 .15 -.15])
  Sec. path : DiscreteFir  Commented=through  Coefficients=[0.5 0.5 -.3 -.3 -.2 -.2]
  Sum : Sum  Inputs=++|
  y : Outport
  wires:
  Primary path/1 -> Sum/2  "Noise output (no ANC)"
  Gain/1 -> y/1, Sec. path/1
  Constant/1 -> LMS Update/3
  LMS filter copy/1 -> Gain/1
  [coefs] -> LMS filter copy/2
  Sum/1 -> LMS Update/2  "Error mic."
  Delay1/1 -> [coefs]
  LMS Update/1 -> Delay1/1
  In1/1 -> Primary path/1, Estim. sec. path/1, LMS filter copy/1
  Estim. sec. path/1 -> LMS Update/1
  Sec. path/1 -> Sum/1

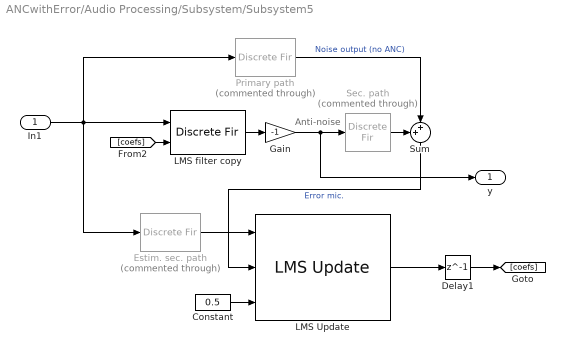
== system ANCwithError/Audio Processing/Subsystem/Subsystem5 ==
  note: Anti-noise
  In1 : Inport
  Constant : Constant  Value=0.5
  Delay1 : Delay  DelayLength=1
  Estim. sec. path : DiscreteFir  Commented=through  Coefficients="[0.466  0.533  -0.257  -0.274  -0.231  -0.175]"
  Gain : Gain  Gain=-1
  LMS Update : dspadpt3/LMS Update  Method=Normalized LMS  Length=200  NumFilters=1  StepSizeSource=Input port  StepSize=0.1  LeakageFactor=1.0  InitialConditions=0  AdaptiveFilterMode=Tapped delay-line FIR filter  EnableAdaptInput=off  EnableResetInput=off  SimulateUsing=Interpreted execution
  LMS filter copy : DiscreteFir  CoefSource=Input port
      settings: InputPortMap=u0,u1
  Primary path : DiscreteFir  Commented=through  Coefficients=conv([0.5 0.5 -.3 -.3 -.2 -.2],[.1 -.1 .2 -.2 .3 -.3 .15 -.15])
  Sec. path : DiscreteFir  Commented=through  Coefficients=[0.5 0.5 -.3 -.3 -.2 -.2]
  Sum : Sum  Inputs=++|
  y : Outport
  wires:
  Primary path/1 -> Sum/2  "Noise output (no ANC)"
  Gain/1 -> y/1, Sec. path/1
  Constant/1 -> LMS Update/3
  LMS filter copy/1 -> Gain/1
  [coefs] -> LMS filter copy/2
  Sum/1 -> LMS Update/2  "Error mic."
  Delay1/1 -> [coefs]
  LMS Update/1 -> Delay1/1
  In1/1 -> Primary path/1, Estim. sec. path/1, LMS filter copy/1
  Estim. sec. path/1 -> LMS Update/1
  Sec. path/1 -> Sum/1

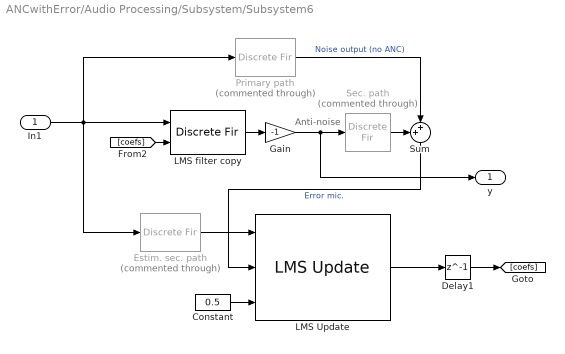
== system ANCwithError/Audio Processing/Subsystem/Subsystem6 ==
  note: Anti-noise
  In1 : Inport
  Constant : Constant  Value=0.5
  Delay1 : Delay  DelayLength=1
  Estim. sec. path : DiscreteFir  Commented=through  Coefficients="[0.466  0.533  -0.257  -0.274  -0.231  -0.175]"
  Gain : Gain  Gain=-1
  LMS Update : dspadpt3/LMS Update  Method=Normalized LMS  Length=200  NumFilters=1  StepSizeSource=Input port  StepSize=0.1  LeakageFactor=1.0  InitialConditions=0  AdaptiveFilterMode=Tapped delay-line FIR filter  EnableAdaptInput=off  EnableResetInput=off  SimulateUsing=Interpreted execution
  LMS filter copy : DiscreteFir  CoefSource=Input port
      settings: InputPortMap=u0,u1
  Primary path : DiscreteFir  Commented=through  Coefficients=conv([0.5 0.5 -.3 -.3 -.2 -.2],[.1 -.1 .2 -.2 .3 -.3 .15 -.15])
  Sec. path : DiscreteFir  Commented=through  Coefficients=[0.5 0.5 -.3 -.3 -.2 -.2]
  Sum : Sum  Inputs=++|
  y : Outport
  wires:
  Primary path/1 -> Sum/2  "Noise output (no ANC)"
  Gain/1 -> y/1, Sec. path/1
  Constant/1 -> LMS Update/3
  LMS filter copy/1 -> Gain/1
  [coefs] -> LMS filter copy/2
  Sum/1 -> LMS Update/2  "Error mic."
  Delay1/1 -> [coefs]
  LMS Update/1 -> Delay1/1
  In1/1 -> Primary path/1, Estim. sec. path/1, LMS filter copy/1
  Estim. sec. path/1 -> LMS Update/1
  Sec. path/1 -> Sum/1

== system ANCwithError/Audio Processing/Subsystem/Subsystem7 ==
  note: Anti-noise
  In1 : Inport
  Constant : Constant  Value=0.5
  Delay1 : Delay  DelayLength=1
  Estim. sec. path : DiscreteFir  Commented=through  Coefficients="[0.466  0.533  -0.257  -0.274  -0.231  -0.175]"
  Gain : Gain  Gain=-1
  LMS Update : dspadpt3/LMS Update  Method=Normalized LMS  Length=200  NumFilters=1  StepSizeSource=Input port  StepSize=0.1  LeakageFactor=1.0  InitialConditions=0  AdaptiveFilterMode=Tapped delay-line FIR filter  EnableAdaptInput=off  EnableResetInput=off  SimulateUsing=Interpreted execution
  LMS filter copy : DiscreteFir  CoefSource=Input port
      settings: InputPortMap=u0,u1
  Primary path : DiscreteFir  Commented=through  Coefficients=conv([0.5 0.5 -.3 -.3 -.2 -.2],[.1 -.1 .2 -.2 .3 -.3 .15 -.15])
  Sec. path : DiscreteFir  Commented=through  Coefficients=[0.5 0.5 -.3 -.3 -.2 -.2]
  Sum : Sum  Inputs=++|
  y : Outport
  wires:
  Primary path/1 -> Sum/2  "Noise output (no ANC)"
  Gain/1 -> y/1, Sec. path/1
  Constant/1 -> LMS Update/3
  LMS filter copy/1 -> Gain/1
  [coefs] -> LMS filter copy/2
  Sum/1 -> LMS Update/2  "Error mic."
  Delay1/1 -> [coefs]
  LMS Update/1 -> Delay1/1
  In1/1 -> Primary path/1, Estim. sec. path/1, LMS filter copy/1
  Estim. sec. path/1 -> LMS Update/1
  Sec. path/1 -> Sum/1

== system ANCwithError/Audio Processing/Subsystem/Subsystem8 ==
  note: Anti-noise
  In1 : Inport
  Constant : Constant  Value=0.5
  Delay1 : Delay  DelayLength=1
  Estim. sec. path : DiscreteFir  Commented=through  Coefficients="[0.466  0.533  -0.257  -0.274  -0.231  -0.175]"
  Gain : Gain  Gain=-1
  LMS Update : dspadpt3/LMS Update  Method=Normalized LMS  Length=200  NumFilters=1  StepSizeSource=Input port  StepSize=0.1  LeakageFactor=1.0  InitialConditions=0  AdaptiveFilterMode=Tapped delay-line FIR filter  EnableAdaptInput=off  EnableResetInput=off  SimulateUsing=Interpreted execution
  LMS filter copy : DiscreteFir  CoefSource=Input port
      settings: InputPortMap=u0,u1
  Primary path : DiscreteFir  Commented=through  Coefficients=conv([0.5 0.5 -.3 -.3 -.2 -.2],[.1 -.1 .2 -.2 .3 -.3 .15 -.15])
  Sec. path : DiscreteFir  Commented=through  Coefficients=[0.5 0.5 -.3 -.3 -.2 -.2]
  Sum : Sum  Inputs=++|
  y : Outport
  wires:
  Primary path/1 -> Sum/2  "Noise output (no ANC)"
  Gain/1 -> y/1, Sec. path/1
  Constant/1 -> LMS Update/3
  LMS filter copy/1 -> Gain/1
  [coefs] -> LMS filter copy/2
  Sum/1 -> LMS Update/2  "Error mic."
  Delay1/1 -> [coefs]
  LMS Update/1 -> Delay1/1
  In1/1 -> Primary path/1, Estim. sec. path/1, LMS filter copy/1
  Estim. sec. path/1 -> LMS Update/1
  Sec. path/1 -> Sum/1

== system ANCwithError/Audio Processing/Subsystem/Subsystem9 ==
  note: Anti-noise
  In1 : Inport
  Constant : Constant  Value=0.5
  Delay1 : Delay  DelayLength=1
  Estim. sec. path : DiscreteFir  Commented=through  Coefficients="[0.466  0.533  -0.257  -0.274  -0.231  -0.175]"
  Gain : Gain  Gain=-1
  LMS Update : dspadpt3/LMS Update  Method=Normalized LMS  Length=200  NumFilters=1  StepSizeSource=Input port  StepSize=0.1  LeakageFactor=1.0  InitialConditions=0  AdaptiveFilterMode=Tapped delay-line FIR filter  EnableAdaptInput=off  EnableResetInput=off  SimulateUsing=Interpreted execution
  LMS filter copy : DiscreteFir  CoefSource=Input port
      settings: InputPortMap=u0,u1
  Primary path : DiscreteFir  Commented=through  Coefficients=conv([0.5 0.5 -.3 -.3 -.2 -.2],[.1 -.1 .2 -.2 .3 -.3 .15 -.15])
  Sec. path : DiscreteFir  Commented=through  Coefficients=[0.5 0.5 -.3 -.3 -.2 -.2]
  Sum : Sum  Inputs=++|
  y : Outport
  wires:
  Primary path/1 -> Sum/2  "Noise output (no ANC)"
  Gain/1 -> y/1, Sec. path/1
  Constant/1 -> LMS Update/3
  LMS filter copy/1 -> Gain/1
  [coefs] -> LMS filter copy/2
  Sum/1 -> LMS Update/2  "Error mic."
  Delay1/1 -> [coefs]
  LMS Update/1 -> Delay1/1
  In1/1 -> Primary path/1, Estim. sec. path/1, LMS filter copy/1
  Estim. sec. path/1 -> LMS Update/1
  Sec. path/1 -> Sum/1

== system ANCwithError/Audio Processing/Subsystem1/Subsystem ==
  note: Anti-noise
  In1 : Inport
  In2 : Inport  Port=2
  Constant : Constant  Value=0.5
  Delay1 : Delay  DelayLength=1
  Estim. sec. path : DiscreteFir  Commented=through  Coefficients="[0.466  0.533  -0.257  -0.274  -0.231  -0.175]"
  Gain : Gain  Gain=-1
  LMS Update : dspadpt3/LMS Update  Method=Normalized LMS  Length=200  NumFilters=1  StepSizeSource=Input port  StepSize=0.1  LeakageFactor=1.0  InitialConditions=0  AdaptiveFilterMode=Tapped delay-line FIR filter  EnableAdaptInput=off  EnableResetInput=off  SimulateUsing=Interpreted execution
  LMS filter copy : DiscreteFir  CoefSource=Input port
      settings: InputPortMap=u0,u1
  y : Outport
  wires:
  Gain/1 -> y/1
  Constant/1 -> LMS Update/3
  LMS filter copy/1 -> Gain/1
  [coefs] -> LMS filter copy/2
  Delay1/1 -> [coefs]
  LMS Update/1 -> Delay1/1
  In1/1 -> Estim. sec. path/1, LMS filter copy/1
  Estim. sec. path/1 -> LMS Update/1
  In2/1 -> LMS Update/2

== system ANCwithError/Audio Processing/Subsystem1/Subsystem1 ==
  In1 : Inport
  In2 : Inport  Port=2
  Constant : Constant  Value=0.5
  Delay1 : Delay  DelayLength=1
  Estim. sec. path : DiscreteFir  Commented=through  Coefficients="[0.466  0.533  -0.257  -0.274  -0.231  -0.175]"
  Gain : Gain  Gain=-1
  LMS Update : dspadpt3/LMS Update  Method=Normalized LMS  Length=200  NumFilters=1  StepSizeSource=Input port  StepSize=0.1  LeakageFactor=1.0  InitialConditions=0  AdaptiveFilterMode=Tapped delay-line FIR filter  EnableAdaptInput=off  EnableResetInput=off  SimulateUsing=Interpreted execution
  LMS filter copy : DiscreteFir  CoefSource=Input port
      settings: InputPortMap=u0,u1
  y : Outport
  wires:
  Gain/1 -> y/1
  Constant/1 -> LMS Update/3
  LMS filter copy/1 -> Gain/1
  [coefs] -> LMS filter copy/2
  Delay1/1 -> [coefs]
  LMS Update/1 -> Delay1/1
  In1/1 -> Estim. sec. path/1, LMS filter copy/1
  Estim. sec. path/1 -> LMS Update/1
  In2/1 -> LMS Update/2

== system ANCwithError/Audio Processing/Subsystem1/Subsystem2 ==
  In1 : Inport
  In2 : Inport  Port=2
  Constant : Constant  Value=0.5
  Delay1 : Delay  DelayLength=1
  Estim. sec. path : DiscreteFir  Commented=through  Coefficients="[0.466  0.533  -0.257  -0.274  -0.231  -0.175]"
  Gain : Gain  Gain=-1
  LMS Update : dspadpt3/LMS Update  Method=Normalized LMS  Length=200  NumFilters=1  StepSizeSource=Input port  StepSize=0.1  LeakageFactor=1.0  InitialConditions=0  AdaptiveFilterMode=Tapped delay-line FIR filter  EnableAdaptInput=off  EnableResetInput=off  SimulateUsing=Interpreted execution
  LMS filter copy : DiscreteFir  CoefSource=Input port
      settings: InputPortMap=u0,u1
  y : Outport
  wires:
  Gain/1 -> y/1
  Constant/1 -> LMS Update/3
  LMS filter copy/1 -> Gain/1
  [coefs] -> LMS filter copy/2
  Delay1/1 -> [coefs]
  LMS Update/1 -> Delay1/1
  In1/1 -> Estim. sec. path/1, LMS filter copy/1
  Estim. sec. path/1 -> LMS Update/1
  In2/1 -> LMS Update/2

== system ANCwithError/Audio Processing/Subsystem1/Subsystem3 ==
  In1 : Inport
  In2 : Inport  Port=2
  Constant : Constant  Value=0.5
  Delay1 : Delay  DelayLength=1
  Estim. sec. path : DiscreteFir  Commented=through  Coefficients="[0.466  0.533  -0.257  -0.274  -0.231  -0.175]"
  Gain : Gain  Gain=-1
  LMS Update : dspadpt3/LMS Update  Method=Normalized LMS  Length=200  NumFilters=1  StepSizeSource=Input port  StepSize=0.1  LeakageFactor=1.0  InitialConditions=0  AdaptiveFilterMode=Tapped delay-line FIR filter  EnableAdaptInput=off  EnableResetInput=off  SimulateUsing=Interpreted execution
  LMS filter copy : DiscreteFir  CoefSource=Input port
      settings: InputPortMap=u0,u1
  y : Outport
  wires:
  Gain/1 -> y/1
  Constant/1 -> LMS Update/3
  LMS filter copy/1 -> Gain/1
  [coefs] -> LMS filter copy/2
  Delay1/1 -> [coefs]
  LMS Update/1 -> Delay1/1
  In1/1 -> Estim. sec. path/1, LMS filter copy/1
  Estim. sec. path/1 -> LMS Update/1
  In2/1 -> LMS Update/2

== system ANCwithError/Audio Processing/Subsystem1/Subsystem4 ==
  In1 : Inport
  In2 : Inport  Port=2
  Constant : Constant  Value=0.5
  Delay1 : Delay  DelayLength=1
  Estim. sec. path : DiscreteFir  Commented=through  Coefficients="[0.466  0.533  -0.257  -0.274  -0.231  -0.175]"
  Gain : Gain  Gain=-1
  LMS Update : dspadpt3/LMS Update  Method=Normalized LMS  Length=200  NumFilters=1  StepSizeSource=Input port  StepSize=0.1  LeakageFactor=1.0  InitialConditions=0  AdaptiveFilterMode=Tapped delay-line FIR filter  EnableAdaptInput=off  EnableResetInput=off  SimulateUsing=Interpreted execution
  LMS filter copy : DiscreteFir  CoefSource=Input port
      settings: InputPortMap=u0,u1
  y : Outport
  wires:
  Gain/1 -> y/1
  Constant/1 -> LMS Update/3
  LMS filter copy/1 -> Gain/1
  [coefs] -> LMS filter copy/2
  Delay1/1 -> [coefs]
  LMS Update/1 -> Delay1/1
  In1/1 -> Estim. sec. path/1, LMS filter copy/1
  Estim. sec. path/1 -> LMS Update/1
  In2/1 -> LMS Update/2

== system ANCwithError/Audio Processing/Subsystem1/Subsystem5 ==
  In1 : Inport
  In2 : Inport  Port=2
  Constant : Constant  Value=0.5
  Delay1 : Delay  DelayLength=1
  Estim. sec. path : DiscreteFir  Commented=through  Coefficients="[0.466  0.533  -0.257  -0.274  -0.231  -0.175]"
  Gain : Gain  Gain=-1
  LMS Update : dspadpt3/LMS Update  Method=Normalized LMS  Length=200  NumFilters=1  StepSizeSource=Input port  StepSize=0.1  LeakageFactor=1.0  InitialConditions=0  AdaptiveFilterMode=Tapped delay-line FIR filter  EnableAdaptInput=off  EnableResetInput=off  SimulateUsing=Interpreted execution
  LMS filter copy : DiscreteFir  CoefSource=Input port
      settings: InputPortMap=u0,u1
  y : Outport
  wires:
  Gain/1 -> y/1
  Constant/1 -> LMS Update/3
  LMS filter copy/1 -> Gain/1
  [coefs] -> LMS filter copy/2
  Delay1/1 -> [coefs]
  LMS Update/1 -> Delay1/1
  In1/1 -> Estim. sec. path/1, LMS filter copy/1
  Estim. sec. path/1 -> LMS Update/1
  In2/1 -> LMS Update/2

== system ANCwithError/Audio Processing/Subsystem1/Subsystem6 ==
  In1 : Inport
  In2 : Inport  Port=2
  Constant : Constant  Value=0.5
  Delay1 : Delay  DelayLength=1
  Estim. sec. path : DiscreteFir  Commented=through  Coefficients="[0.466  0.533  -0.257  -0.274  -0.231  -0.175]"
  Gain : Gain  Gain=-1
  LMS Update : dspadpt3/LMS Update  Method=Normalized LMS  Length=200  NumFilters=1  StepSizeSource=Input port  StepSize=0.1  LeakageFactor=1.0  InitialConditions=0  AdaptiveFilterMode=Tapped delay-line FIR filter  EnableAdaptInput=off  EnableResetInput=off  SimulateUsing=Interpreted execution
  LMS filter copy : DiscreteFir  CoefSource=Input port
      settings: InputPortMap=u0,u1
  y : Outport
  wires:
  Gain/1 -> y/1
  Constant/1 -> LMS Update/3
  LMS filter copy/1 -> Gain/1
  [coefs] -> LMS filter copy/2
  Delay1/1 -> [coefs]
  LMS Update/1 -> Delay1/1
  In1/1 -> Estim. sec. path/1, LMS filter copy/1
  Estim. sec. path/1 -> LMS Update/1
  In2/1 -> LMS Update/2

== system ANCwithError/Audio Processing/Subsystem1/Subsystem7 ==
  note: Anti-noise
  In1 : Inport
  In2 : Inport  Port=2
  Constant : Constant  Value=0.5
  Delay1 : Delay  DelayLength=1
  Estim. sec. path : DiscreteFir  Commented=through  Coefficients="[0.466  0.533  -0.257  -0.274  -0.231  -0.175]"
  Gain : Gain  Gain=-1
  LMS Update : dspadpt3/LMS Update  Method=Normalized LMS  Length=200  NumFilters=1  StepSizeSource=Input port  StepSize=0.1  LeakageFactor=1.0  InitialConditions=0  AdaptiveFilterMode=Tapped delay-line FIR filter  EnableAdaptInput=off  EnableResetInput=off  SimulateUsing=Interpreted execution
  LMS filter copy : DiscreteFir  CoefSource=Input port
      settings: InputPortMap=u0,u1
  y : Outport
  wires:
  Gain/1 -> y/1
  Constant/1 -> LMS Update/3
  LMS filter copy/1 -> Gain/1
  [coefs] -> LMS filter copy/2
  Delay1/1 -> [coefs]
  LMS Update/1 -> Delay1/1
  In1/1 -> Estim. sec. path/1, LMS filter copy/1
  Estim. sec. path/1 -> LMS Update/1
  In2/1 -> LMS Update/2

== system ANCwithError/Audio Processing/Subsystem1/Subsystem8 ==
  note: Anti-noise
  In1 : Inport
  In2 : Inport  Port=2
  Constant : Constant  Value=0.5
  Delay1 : Delay  DelayLength=1
  Estim. sec. path : DiscreteFir  Commented=through  Coefficients="[0.466  0.533  -0.257  -0.274  -0.231  -0.175]"
  Gain : Gain  Gain=-1
  LMS Update : dspadpt3/LMS Update  Method=Normalized LMS  Length=200  NumFilters=1  StepSizeSource=Input port  StepSize=0.1  LeakageFactor=1.0  InitialConditions=0  AdaptiveFilterMode=Tapped delay-line FIR filter  EnableAdaptInput=off  EnableResetInput=off  SimulateUsing=Interpreted execution
  LMS filter copy : DiscreteFir  CoefSource=Input port
      settings: InputPortMap=u0,u1
  y : Outport
  wires:
  Gain/1 -> y/1
  Constant/1 -> LMS Update/3
  LMS filter copy/1 -> Gain/1
  [coefs] -> LMS filter copy/2
  Delay1/1 -> [coefs]
  LMS Update/1 -> Delay1/1
  In1/1 -> Estim. sec. path/1, LMS filter copy/1
  Estim. sec. path/1 -> LMS Update/1
  In2/1 -> LMS Update/2

== system ANCwithError/Audio Processing/Subsystem1/Subsystem9 ==
  note: Anti-noise
  In1 : Inport
  In2 : Inport  Port=2
  Constant : Constant  Value=0.5
  Delay1 : Delay  DelayLength=1
  Estim. sec. path : DiscreteFir  Commented=through  Coefficients="[0.466  0.533  -0.257  -0.274  -0.231  -0.175]"
  Gain : Gain  Gain=-1
  LMS Update : dspadpt3/LMS Update  Method=Normalized LMS  Length=200  NumFilters=1  StepSizeSource=Input port  StepSize=0.1  LeakageFactor=1.0  InitialConditions=0  AdaptiveFilterMode=Tapped delay-line FIR filter  EnableAdaptInput=off  EnableResetInput=off  SimulateUsing=Interpreted execution
  LMS filter copy : DiscreteFir  CoefSource=Input port
      settings: InputPortMap=u0,u1
  y : Outport
  wires:
  Gain/1 -> y/1
  Constant/1 -> LMS Update/3
  LMS filter copy/1 -> Gain/1
  [coefs] -> LMS filter copy/2
  Delay1/1 -> [coefs]
  LMS Update/1 -> Delay1/1
  In1/1 -> Estim. sec. path/1, LMS filter copy/1
  Estim. sec. path/1 -> LMS Update/1
  In2/1 -> LMS Update/2

== system ANCwithError/Audio Processing/Subsystem2/Subsystem ==
  note: Anti-noise
  In1 : Inport
  In2 : Inport  Port=2
  Constant : Constant  Value=0.5
  Delay1 : Delay  DelayLength=1
  Estim. sec. path : DiscreteFir  Commented=through  Coefficients="[0.466  0.533  -0.257  -0.274  -0.231  -0.175]"
  Gain : Gain  Gain=-1
  LMS Update : dspadpt3/LMS Update  Method=Normalized LMS  Length=200  NumFilters=1  StepSizeSource=Input port  StepSize=0.1  LeakageFactor=1.0  InitialConditions=0  AdaptiveFilterMode=Tapped delay-line FIR filter  EnableAdaptInput=off  EnableResetInput=off  SimulateUsing=Interpreted execution
  LMS filter copy : DiscreteFir  CoefSource=Input port
      settings: InputPortMap=u0,u1
  y : Outport
  wires:
  Gain/1 -> y/1
  Constant/1 -> LMS Update/3
  LMS filter copy/1 -> Gain/1
  [coefs] -> LMS filter copy/2
  Delay1/1 -> [coefs]
  LMS Update/1 -> Delay1/1
  In1/1 -> Estim. sec. path/1, LMS filter copy/1
  Estim. sec. path/1 -> LMS Update/1
  In2/1 -> LMS Update/2

== system ANCwithError/Audio Processing/Subsystem2/Subsystem1 ==
  In1 : Inport
  In2 : Inport  Port=2
  Constant : Constant  Value=0.5
  Delay1 : Delay  DelayLength=1
  Estim. sec. path : DiscreteFir  Commented=through  Coefficients="[0.466  0.533  -0.257  -0.274  -0.231  -0.175]"
  Gain : Gain  Gain=-1
  LMS Update : dspadpt3/LMS Update  Method=Normalized LMS  Length=200  NumFilters=1  StepSizeSource=Input port  StepSize=0.1  LeakageFactor=1.0  InitialConditions=0  AdaptiveFilterMode=Tapped delay-line FIR filter  EnableAdaptInput=off  EnableResetInput=off  SimulateUsing=Interpreted execution
  LMS filter copy : DiscreteFir  CoefSource=Input port
      settings: InputPortMap=u0,u1
  y : Outport
  wires:
  Gain/1 -> y/1
  Constant/1 -> LMS Update/3
  LMS filter copy/1 -> Gain/1
  [coefs] -> LMS filter copy/2
  Delay1/1 -> [coefs]
  LMS Update/1 -> Delay1/1
  In1/1 -> Estim. sec. path/1, LMS filter copy/1
  Estim. sec. path/1 -> LMS Update/1
  In2/1 -> LMS Update/2

== system ANCwithError/Audio Processing/Subsystem2/Subsystem2 ==
  In1 : Inport
  In2 : Inport  Port=2
  Constant : Constant  Value=0.5
  Delay1 : Delay  DelayLength=1
  Estim. sec. path : DiscreteFir  Commented=through  Coefficients="[0.466  0.533  -0.257  -0.274  -0.231  -0.175]"
  Gain : Gain  Gain=-1
  LMS Update : dspadpt3/LMS Update  Method=Normalized LMS  Length=200  NumFilters=1  StepSizeSource=Input port  StepSize=0.1  LeakageFactor=1.0  InitialConditions=0  AdaptiveFilterMode=Tapped delay-line FIR filter  EnableAdaptInput=off  EnableResetInput=off  SimulateUsing=Interpreted execution
  LMS filter copy : DiscreteFir  CoefSource=Input port
      settings: InputPortMap=u0,u1
  y : Outport
  wires:
  Gain/1 -> y/1
  Constant/1 -> LMS Update/3
  LMS filter copy/1 -> Gain/1
  [coefs] -> LMS filter copy/2
  Delay1/1 -> [coefs]
  LMS Update/1 -> Delay1/1
  In1/1 -> Estim. sec. path/1, LMS filter copy/1
  Estim. sec. path/1 -> LMS Update/1
  In2/1 -> LMS Update/2

== system ANCwithError/Audio Processing/Subsystem2/Subsystem3 ==
  In1 : Inport
  In2 : Inport  Port=2
  Constant : Constant  Value=0.5
  Delay1 : Delay  DelayLength=1
  Estim. sec. path : DiscreteFir  Commented=through  Coefficients="[0.466  0.533  -0.257  -0.274  -0.231  -0.175]"
  Gain : Gain  Gain=-1
  LMS Update : dspadpt3/LMS Update  Method=Normalized LMS  Length=200  NumFilters=1  StepSizeSource=Input port  StepSize=0.1  LeakageFactor=1.0  InitialConditions=0  AdaptiveFilterMode=Tapped delay-line FIR filter  EnableAdaptInput=off  EnableResetInput=off  SimulateUsing=Interpreted execution
  LMS filter copy : DiscreteFir  CoefSource=Input port
      settings: InputPortMap=u0,u1
  y : Outport
  wires:
  Gain/1 -> y/1
  Constant/1 -> LMS Update/3
  LMS filter copy/1 -> Gain/1
  [coefs] -> LMS filter copy/2
  Delay1/1 -> [coefs]
  LMS Update/1 -> Delay1/1
  In1/1 -> Estim. sec. path/1, LMS filter copy/1
  Estim. sec. path/1 -> LMS Update/1
  In2/1 -> LMS Update/2
